simulink model "bezRegulatora"  (R2019b)
settings: Solver=VariableStepAuto  StartTime=0.0  StopTime=40  RelTol=1e-3
values from neighbouring files (symbols this model uses):
  k = str2num(answer{1,1})    [index.m]
  numerWybranegoWymuszenia = menu('Wybierz wymuszenie', 'wymuszenie skokowe u(t)=1(t-10)', 'wymuszenie pulsowe u(t)=1(t-10)-1(t-11)')    [index.m]
  T0 = str2num(answer{7,1})    [index.m]
  T1 = str2num(answer{2,1})    [index.m]
  T2 = str2num(answer{3,1})    [index.m]
  T3 = str2num(answer{4,1})    [index.m]
  T4 = str2num(answer{5,1})    [index.m]
  T5 = str2num(answer{6,1})    [index.m]
settings Model: Creator=01129847  LastModifiedBy=01129847

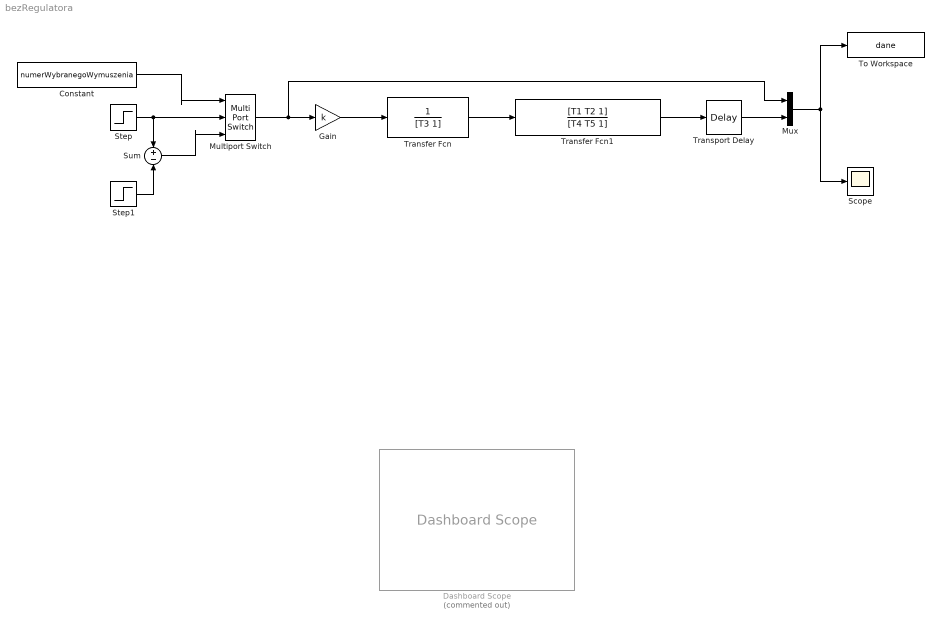
== system bezRegulatora ==
  Constant : Constant  Value=numerWybranegoWymuszenia
  Dashboard Scope : DashboardScope  Commented=on
  Gain : Gain  Gain=k
  Multiport Switch : MultiPortSwitch  Inputs=2
  Mux : Mux  Inputs=2
  Scope : Scope
  Step : Step  Time=10  SampleTime=0
  Step1 : Step  Time=11  SampleTime=0
  Sum : Sum  Inputs=+-
  To Workspace : ToWorkspace  VariableName=dane  SaveFormat=Timeseries  SampleTime=0.1
      settings: Save2DSignal=2-D array (concatenate along first dimension)
  Transfer Fcn : TransferFcn  Denominator=[T3 1]
  Transfer Fcn1 : TransferFcn  Numerator=[T1 T2 1]  Denominator=[T4 T5 1]
  Transport Delay : TransportDelay  DelayTime=T0
  wires:
  Multiport Switch/1 -> Mux/1, Gain/1
  Gain/1 -> Transfer Fcn/1
  Transfer Fcn/1 -> Transfer Fcn1/1
  Transfer Fcn1/1 -> Transport Delay/1
  Transport Delay/1 -> Mux/2
  Mux/1 -> To Workspace/1, Scope/1
  Step/1 -> Multiport Switch/2, Sum/1
  Step1/1 -> Sum/2
  Sum/1 -> Multiport Switch/3
  Constant/1 -> Multiport Switch/1
